simulink model "testmodel"  (R2012b)
settings: Solver=ode3  StartTime=0.0  StopTime=10.0  FixedStep=1  RelTol=1e-3
values from neighbouring files (symbols this model uses):
  MFin1 = [-1.8 -0.8 0.2 ... (first row only)    [test_fuzzy.m]
  MFin2 = [-5.4 -2.4 0.6 ... (first row only)    [test_fuzzy.m]
  MFout = [-3.6 -1.6 0.4 ... (first row only)    [test_fuzzy.m]
  R = [1 1 2 ... (first row only)    [test_fuzzy.m]
libraries: fuzblock x1
settings Model: Creator=omaki  LastModifiedBy=omaki
settings DataIOCC: SignalLoggingSaveFormat=ModelDataLogs
settings OptimizationCC: InlineParams=on
settings GRTTargetCC: CombineOutputUpdateFcns=off  GRTInterface=on

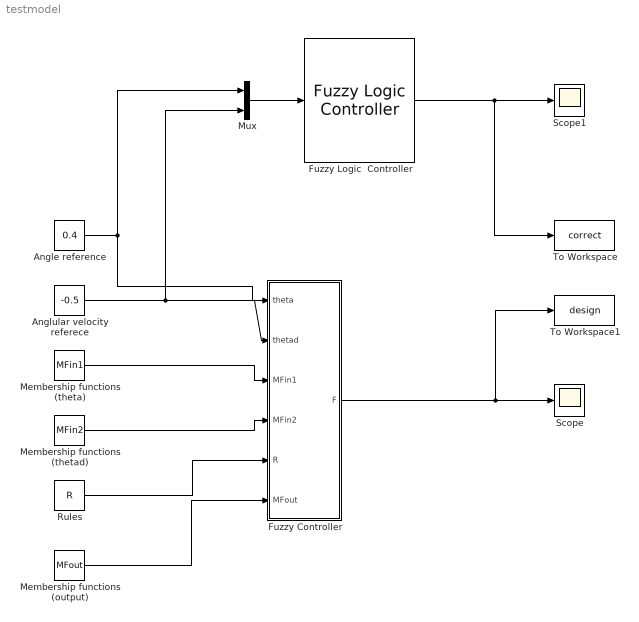
== system testmodel ==
  "Angle reference " : Constant  Value=0.4
  Anglular velocity referece : Constant  Value=-0.5
  Fuzzy Controller : MATLAB Function  TreatAsAtomicUnit=on
  Fuzzy Logic  Controller : fuzblock/Fuzzy Logic  Controller  fis=compare
  Membership functions (output) : Constant  Value=MFout
  Membership functions (theta) : Constant  Value=MFin1
  Membership functions (thetad) : Constant  Value=MFin2
  Mux : Mux  Inputs=2
  Rules : Constant  Value=R
  Scope : Scope
  Scope1 : Scope
  To Workspace : ToWorkspace  VariableName=correct  SampleTime=-1
  To Workspace1 : ToWorkspace  VariableName=design  SampleTime=-1
  wires:
  Membership functions (theta)/1 -> Fuzzy Controller/3(MFin1)
  Membership functions (thetad)/1 -> Fuzzy Controller/4(MFin2)
  Rules/1 -> Fuzzy Controller/5(R)
  Membership functions (output)/1 -> Fuzzy Controller/6(MFout)
  "Angle reference "/1 -> Fuzzy Controller/1(theta), Mux/1
  Anglular velocity referece/1 -> Mux/2, Fuzzy Controller/2(thetad)
  Mux/1 -> Fuzzy Logic  Controller/1
  Fuzzy Logic  Controller/1 -> To Workspace/1, Scope1/1
  Fuzzy Controller/1(F) -> To Workspace1/1, Scope/1

== matlab function testmodel/Fuzzy Controller ==
  data: theta input; F output; thetad input; MFin1 input; MFin2 input; R input; MFout input
function F = fcn(theta, thetad, MFin1, MFin2, R, MFout)
Btheta = calculateBelonging(MFin1, theta);
Bthetad = calculateBelonging(MFin2, thetad);
Bout = applyRules(R, Btheta, Bthetad, MFout);
F = defuzzify(Bout, MFout);
